simulink model "dcm_compatible"  (R2021a)
settings: Solver=ode1  StartTime=0.0  StopTime=33  FixedStep=Ts  RelTol=1e-3
undefined symbols (not defined in the file or in its folder): National_Instruments, PCIe
libraries: sldrtlib x2, simulink x1
Description:
  | Water Tank Model with Dashboard
  | 
  | The example model "sldrtex_dashboard" shows a real-time model of a water tank
  | controlled by dashboard controls.  You can change the inputs to the plant using
  | the knobs and observe the response on the gauges.
  | 
  | How to run this model in Normal Mode:
  | 
  | 1) Double-click the orange button to switch to Normal Mode if needed.
  | 2) Start the real-time execution using Simulation->Run.
  | 3) Change the input flow and output valve values by the dashboard controls and observe
  |    the results on the dashboard gauges.
  | 
  | How to run this model in External Mode:
  | 
  | 1) Double-click the orange button to switch to External Mode if needed.
  | 2) Start the real-time execution using Simulation->Run. The model will automatically
  |    build, connect to Simulink in External Mode and start.
  | 3) Change the input flow and output valve values by the dashboard controls and observe
  |    the results on the dashboard gauges.
settings Model: SimulationMode=external  ExtModeTrigDuration=100001  Creator=The MathWorks, Inc.  LastModifiedBy=parida
settings SolverCC: AlgebraicLoopSolver=TrustRegion  AutoInsertRateTranBlk=on
settings DataIOCC: LimitDataPoints=on  SaveFormat=Array  ReturnWorkspaceOutputs=off  SignalLoggingName=logsOut
settings OptimizationCC: ExpressionDepthLimit=2147483647  InitFltsAndDblsToZero=on  EfficientMapNaN2IntZero=off  LifeSpan=inf
settings DebuggingCC: UnderspecifiedInitializationDetection=Classic  MergeDetectMultiDrivingBlocksExec=none  SignalResolutionControl=TryResolveAllWithWarning  FcnCallInpInsideContextMsg=warning  AllowSymbolicDim=off  StateNameClashWarn=warning  SFUnexpectedBacktrackingDiag=warning  SFNoUnconditionalDefaultTransitionDiag=warning  SFExecutionAtInitializationDiag=none  ArithmeticOperatorsInVariantConditions=warning
settings HardwareCC: TargetBitPerLong=64  TargetBitPerPointer=64  TargetBitPerSizeT=64  TargetBitPerPtrDiffT=64  TargetIntDivRoundTo=Zero  TargetEndianess=LittleEndian  TargetWordSize=64  TargetHWDeviceType=Intel->x86-64
settings ModelReferenceCC: PropagateSignalLabelsOutOfModel=off
settings SFSimCC: SimUseLocalCustomCode=off  CustomCodeUndefinedFunction=UseInterfaceOnly
settings RTWCC: Description=Simulink Desktop Real-Time  SystemTargetFile=sldrt.tlc  TemplateMakefile=sldrt.tmf  RTWUseLocalCustomCode=off  RTWCompilerOptimization=on
settings CodeAppCC: MaxIdLength=95  StateflowObjectComments=on
settings SimulinkDesktopRealTimeCC: TargetPreCompLibLocation=C:\Program Files\MATLAB\R2021a\toolbox\sldrt\lib\win64  TargetLangStandard=C89/C90 (ANSI)  SupportVariableSizeSignals=off
settings ConfigComp: CovMetricSettings=dw  CovSaveCumulativeToWorkspaceVar=on  CovSaveSingleToWorkspaceVar=on  CovExternalEMLEnable=off  CovSFcnEnable=off

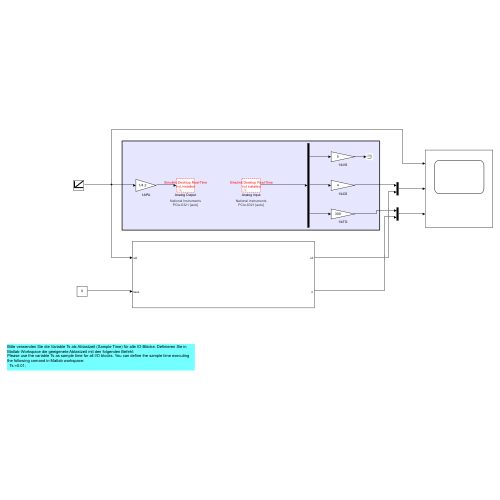
[thumbnail: Simulink's stored preview of the top-level diagram]
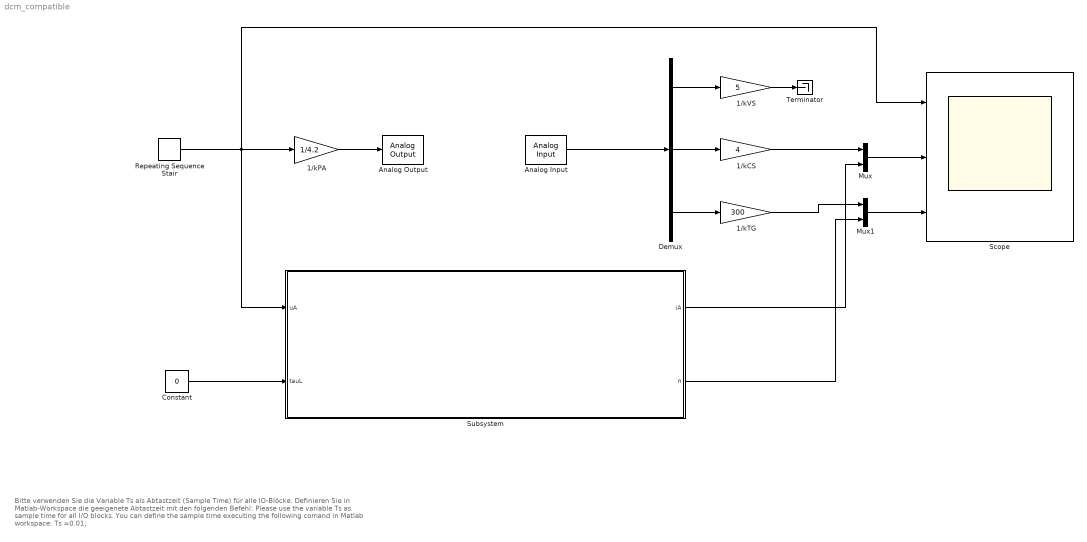
== system dcm_compatible ==
  note: Bitte verwenden Sie die Variable Ts als Abtastzeit (Sample Time) für alle IO-Blöcke. Definieren Sie in Matlab-Workspace die geeigenete Abtastzeit mit den folgenden Befehl:
      | Please use the variable Ts as sample time for all I/O blocks. You can define the sample time executing the following comand in Matlab workspace:
      |   Ts =0.01;
  1/kCS : Gain  Gain=4
  1/kPA : Gain  Gain=1/4.2
  1/kTG : Gain  Gain=300
  1/kVS : Gain  Gain=5
  Analog Input : sldrtlib/Analog Input  SampleTime=0.001  MaxMissedTicks=10  ShowMissedTicks=off  YieldWhenWaiting=off  DrvName=National_Instruments/PCIe-6321  DrvAddress=4294967295  DrvOptions=[0 0 0 0 0 0 0]  Channels=[1 2 3]  RangeMode=1  VoltRange=1  DataType=1
      settings: AttributesFormatString=National Instruments\nPCIe-6321 [auto]
  Analog Output : sldrtlib/Analog Output  SampleTime=0.001  MaxMissedTicks=10  ShowMissedTicks=off  YieldWhenWaiting=off  DrvName=National_Instruments/PCIe-6321  DrvAddress=4294967295  DrvOptions=[0 0 0 0 0 0 0]  Channels=1  RangeMode=1  VoltRange=1  InitialValue=0  FinalValue=0
      settings: AttributesFormatString=National Instruments\nPCIe-6321 [auto]
  Constant : Constant  Value=0
  Demux : Demux  Outputs=3
  Mux : Mux  Inputs=2
  Mux1 : Mux  Inputs=2
  Repeating Sequence Stair : simulink/Sources/Repeating Sequence Stair  OutValues=[0:3:30]  tsamp=3  OutMin=[]  OutMax=[]  OutDataTypeStr=double  OutputDataTypeScalingMode=double  OutDataType=fixdt(0,8)  ConRadixGroup=Best Precision: Vector-wise  OutScaling=2^-12
  Scope : Scope  NumInputPorts=3
  Subsystem : Subsystem
  Terminator : Terminator
  wires:
  Demux/1 -> 1/kVS/1
  Demux/2 -> 1/kCS/1
  Demux/3 -> 1/kTG/1
  1/kPA/1 -> Analog Output/1
  Analog Input/1 -> Demux/1
  1/kVS/1 -> Terminator/1
  Repeating Sequence Stair/1 -> Subsystem/1(uA), Scope/1, 1/kPA/1
  1/kCS/1 -> Mux/1
  1/kTG/1 -> Mux1/1
  Mux/1 -> Scope/2
  Mux1/1 -> Scope/3
  Subsystem/1(iA) -> Mux/2
  Subsystem/2(n) -> Mux1/2
  Constant/1 -> Subsystem/2(tauL)

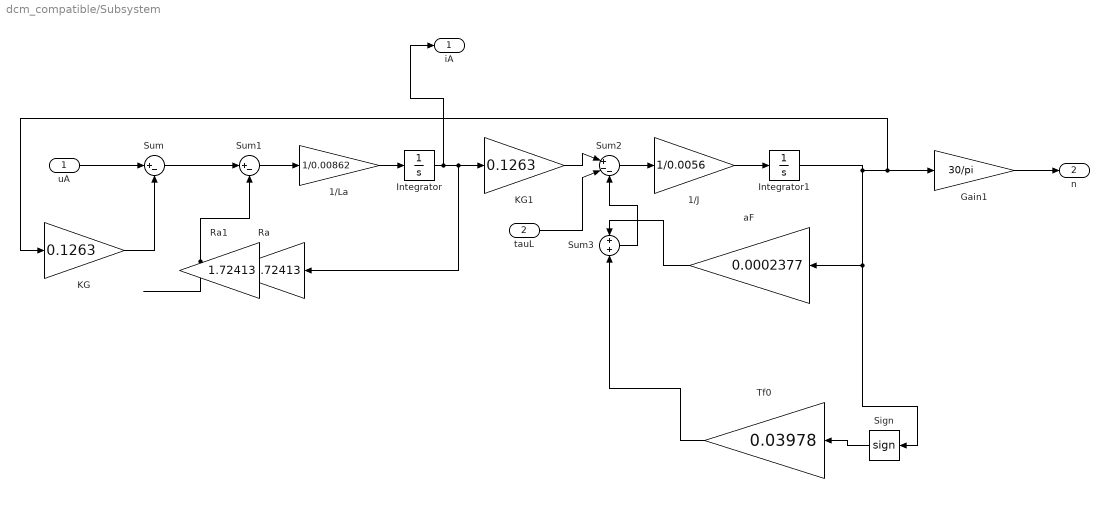
== system dcm_compatible/Subsystem ==
  uA : Inport
  tauL : Inport  Port=2
  1/J : Gain  Gain=1/0.0056
  1/La : Gain  Gain=1/0.00862
  Gain1 : Gain  Gain=30/pi
  Integrator : Integrator
  Integrator1 : Integrator
  KG : Gain  Gain=0.1263
  KG1 : Gain  Gain=0.1263
  Ra : Gain  Gain=1.72413
  Ra1 : Gain  Gain=1.72413
  Sign : Signum
  Sum : Sum  Inputs=|+-
  Sum1 : Sum  Inputs=|+-
  Sum2 : Sum  Inputs=|+--
  Sum3 : Sum  Inputs=+|+
  Tf0 : Gain  Gain=0.03978
  aF : Gain  Gain=0.0002377
  iA : Outport
  n : Outport  Port=2
  wires:
  uA/1 -> Sum/1
  Sum/1 -> Sum1/1
  Sum1/1 -> 1/La/1
  1/La/1 -> Integrator/1
  Ra/1 -> Sum1/2
  Integrator/1 -> KG1/1, Ra/1, iA/1
  KG/1 -> Sum/2
  KG1/1 -> Sum2/1
  tauL/1 -> Sum2/2
  Sum2/1 -> 1/J/1
  1/J/1 -> Integrator1/1
  Gain1/1 -> n/1
  Integrator1/1 -> Sign/1, aF/1, KG/1, Gain1/1
  Tf0/1 -> Sum3/2
  Sum3/1 -> Sum2/3
  aF/1 -> Sum3/1
  Sign/1 -> Tf0/1
